simulink model "Daolibai_design_SFandPIOFtu"  (R2016a)
settings: Solver=VariableStepAuto  SolverMode=SingleTasking  StartTime=0.0  StopTime=50  RelTol=1e-3
values from neighbouring files (symbols this model uses):
  A = [-18/7 9 0;1 -1 1;0 -14.28 0]    [Caishidianlu_design.m]    (also in Daolibai_analysis_ControllAndObserv.m = [0 1 0 0; Daolibai_analysis_stability.m = [0 1 0 0; Daolibai_design_OSF.m = [0 1 0 0; Daolibai_design_OSFandPIOF.m = [0 1 0 0)
  B = [27/7;0;0]    [Caishidianlu_design.m]    (also in Daolibai_analysis_ControllAndObserv.m = [0;1;0;-2]; Daolibai_analysis_stability.m = [0;1;0;-2]; Daolibai_design_OSF.m = [0;1;0;-2]; Daolibai_design_OSFandPIOF.m = [0;1;0;-2])
  C = [1 0 0]    [Caishidianlu_design.m]    (also in Daolibai_analysis_ControllAndObserv.m = [1 0 0 0]; Daolibai_analysis_stability.m = [1 0 0 0]; Daolibai_design_OSF.m = [1 0 0 0]; Daolibai_design_OSFandPIOF.m = [1 0 0 0])
  Init = [0.1 0.1 0.5 0.5]    [Daolibai_design_OSF.m]    (also in Daolibai_design_OSFandPIOF.m = [0 0.04 0.005 0.1 ]; Daolibai_design_SFandOF.m; Daolibai_design_SFandPIOF.m = [0 0.1 0.005 0.1 ])
  K1 = K(:,1:4)    [Daolibai_design_OSFandPIOF.m]    (also in Daolibai_design_SFandPIOF.m)
  K2 = -K(:,5:5)    [Daolibai_design_OSFandPIOF.m]    (also in Daolibai_design_SFandPIOF.m)
settings Model: Creator=19017  LastModifiedBy=19017
settings DataIOCC: ReturnWorkspaceOutputs=on
settings DebuggingCC: SFUnexpectedBacktrackingDiag=error  SFNoUnconditionalDefaultTransitionDiag=error
settings SFSimCC: SimUseLocalCustomCode=on
settings RTWCC: RTWUseLocalCustomCode=on
settings GRTTargetCC: TargetLangStandard=C99 (ISO)
settings ConfigComp: CovMetricSettings=dwe  CovSaveCumulativeToWorkspaceVar=off  CovSaveSingleToWorkspaceVar=off  CovExternalEMLEnable=on

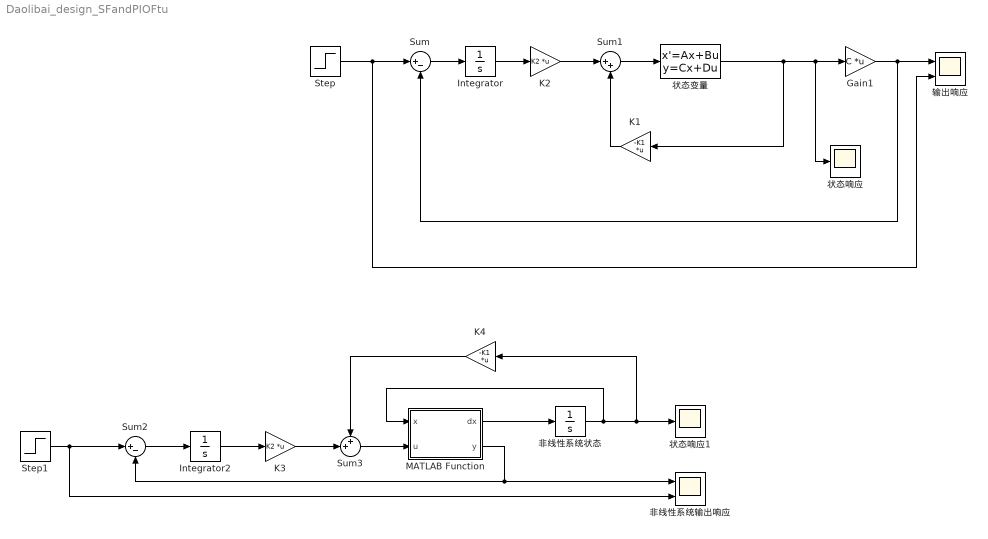
== system Daolibai_design_SFandPIOFtu ==
  Gain1 : Gain  Gain=C  Multiplication=Matrix(K*u)
  Integrator : Integrator  InitialCondition=[0]
  Integrator2 : Integrator  InitialCondition=[0]
  K1 : Gain  Gain=-K1  Multiplication=Matrix(K*u)
  K2 : Gain  Gain=K2  Multiplication=Matrix(K*u)
  K3 : Gain  Gain=K2  Multiplication=Matrix(K*u)
  K4 : Gain  Gain=-K1  Multiplication=Matrix(K*u)
  MATLAB Function : MATLAB Function  TreatAsAtomicUnit=on
  Step : Step  SampleTime=0
  Step1 : Step  SampleTime=0
  Sum : Sum  Inputs=|+-
  Sum1 : Sum  Inputs=|++
  Sum2 : Sum  Inputs=|+-
  Sum3 : Sum  Inputs=++|
  状态变量 : StateSpace  A=A  B=B  C=eye(4)  D=[0;0;0;0]  X0=Init
  状态响应 : Scope
  状态响应1 : Scope
  输出响应 : Scope  NumInputPorts=2
  非线性系统状态 : Integrator  InitialCondition=Init
  非线性系统输出响应 : Scope  NumInputPorts=2
  wires:
  状态变量/1 -> K1/1, 状态响应/1, Gain1/1
  Gain1/1 -> Sum/2, 输出响应/1
  Sum1/1 -> 状态变量/1
  Step/1 -> 输出响应/2, Sum/1
  Sum/1 -> Integrator/1
  Integrator/1 -> K2/1
  K1/1 -> Sum1/2
  K2/1 -> Sum1/1
  MATLAB Function/1(dx) -> 非线性系统状态/1
  非线性系统状态/1 -> 状态响应1/1, K4/1, MATLAB Function/1(x)
  Step1/1 -> 非线性系统输出响应/2, Sum2/1
  Sum2/1 -> Integrator2/1
  Integrator2/1 -> K3/1
  Sum3/1 -> MATLAB Function/2(u)
  K3/1 -> Sum3/2
  K4/1 -> Sum3/1
  MATLAB Function/2(y) -> 非线性系统输出响应/1, Sum2/2

== matlab function Daolibai_design_SFandPIOFtu/MATLAB Function ==
  data: x input; dx output; u input; y output
function [dx,y] = fcn(x,u)
M = 1;
m = 0.1;
l = 0.5;
g = 9.8;
x1=x(1);
x2=x(2);
x3=x(3);
x4=x(4);
dx1 = x2;
dx2 =(u + m*l*x4*x4*sin(x3) - m*g*sin(x3)*cos(x3))/(M + m - m*cos(x3)*cos(x3));
dx3 = x4;
dx4 =(-u*cos(x3) + (M+m)*g*sin(x3) - m*l*x4*x4*sin(x3)*cos(x3))/((M+m)*l - m*l*cos(x3)*cos(x3));
dx = [dx1;dx2;dx3;dx4];
y = x1;
